simulink model "DR_Telemedicine_Screening_Workflow"  (R2024b)
settings: Solver=VariableStepAuto  StartTime=0.0  StopTime=28800  RelTol=1e-3
undefined symbols (not defined in the file): m, n
settings Model: Creator=amrut  LastModifiedBy=amrut

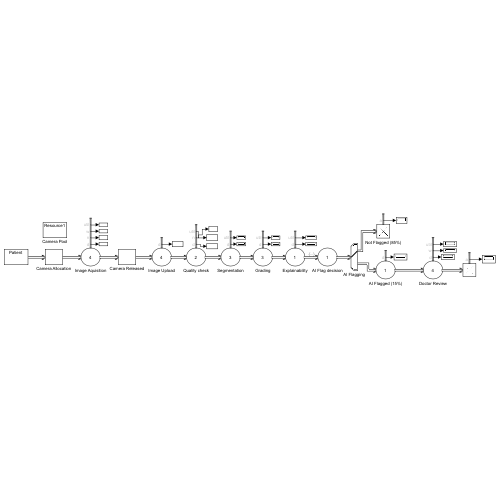
[thumbnail: Simulink's stored preview of the top-level diagram]
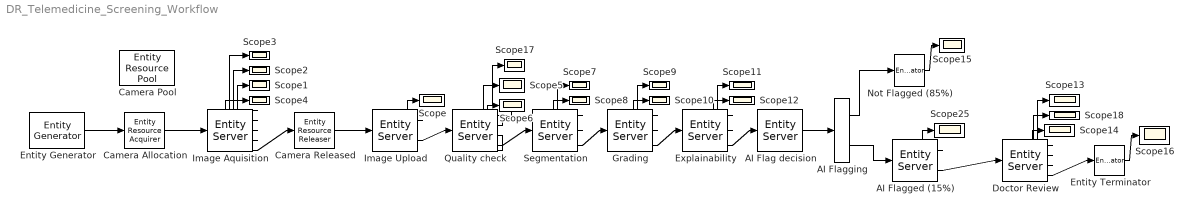
== system DR_Telemedicine_Screening_Workflow ==
  AI Flag decision : EntityServer  InputPortMessageModes=m  OutputPortMessageModes=m  Capacity=1  EntryAction=|
      | if rand < 0.15
      |     entity.Attribute1 = 2;
      | else
      |     entity.Attribute1 = 1;
      | end
  AI Flagged (15%) : EntityServer  InputPortMessageModes=m  OutputPortMessageModes=n,m  Capacity=1  NumberEntitiesDeparted=on
      settings: OutputPortMap=o0,o9
  AI Flagging : EntityOutputSwitch  InputPortMessageModes=m  OutputPortMessageModes=m,m  SwitchingCriterion=From attribute  SwitchAttributeName=Attribute1
  Camera Allocation : EntityResourceAcquirer  InputPortMessageModes=m  OutputPortMessageModes=m  NumberWaitingEntities=inf
      settings: OutputPortMap=o3
  Camera Pool : EntityResourcePool  ResourceAmount=4
  Camera Released : EntityResourceReleaser  InputPortMessageModes=m  OutputPortMessageModes=m  ResourceToRelease=Selected  ResourceAmount=1
  Doctor Review : EntityServer  InputPortMessageModes=m  OutputPortMessageModes=n,n,n,m  Capacity=4  ServiceTimeValue=900  NumberEntitiesDeparted=on  AverageWait=on  Utilization=on
      settings: OutputPortMap=o0,o4,o5,o9
  Entity Generator : EntityGenerator  OutputPortMessageModes=m  Period=86.49  EntityType=Structured  EntityTypeName=Patient
  Entity Terminator : EntityTerminator  InputPortMessageModes=m  NumberEntitiesArrived=on
      settings: OutputPortMap=o0
  Explainability : EntityServer  InputPortMessageModes=m  OutputPortMessageModes=n,n,m  Capacity=1  ServiceTimeValue=30  NumberEntitiesDeparted=on  Utilization=on
      settings: OutputPortMap=o0,o5,o9
  Grading : EntityServer  InputPortMessageModes=m  OutputPortMessageModes=n,n,m  Capacity=3  ServiceTimeValue=60  NumberEntitiesDeparted=on  Utilization=on
      settings: OutputPortMap=o0,o5,o9
  Image Aquisition : EntityServer  InputPortMessageModes=m  OutputPortMessageModes=n,n,n,n,m  Capacity=4  ServiceTimeValue=300  NumberEntitiesDeparted=on  NumberEntitiesInBlock=on  AverageWait=on  Utilization=on
      settings: OutputPortMap=o0,o1,o4,o5,o9
  Image Upload : EntityServer  InputPortMessageModes=m  OutputPortMessageModes=n,m  Capacity=4  ServiceTimeValue=4  NumberEntitiesDeparted=on
      settings: OutputPortMap=o0,o9
  Not Flagged (85%) : EntityTerminator  InputPortMessageModes=m  NumberEntitiesArrived=on
      settings: OutputPortMap=o0
  Quality check : EntityServer  InputPortMessageModes=m  OutputPortMessageModes=n,n,n,m  Capacity=2  ServiceTimeValue=30  NumberEntitiesDeparted=on  NumberEntitiesInBlock=on  Utilization=on
      settings: OutputPortMap=o0,o1,o5,o9
  Scope{,1..18,25} (20 alike) : Scope
  Segmentation : EntityServer  InputPortMessageModes=m  OutputPortMessageModes=n,n,m  Capacity=3  ServiceTimeValue=90  NumberEntitiesDeparted=on  Utilization=on
      settings: OutputPortMap=o0,o5,o9
  wires:
  Entity Generator/1 -> Camera Allocation/1
  Camera Allocation/1 -> Image Aquisition/1
  Image Aquisition/5 -> Camera Released/1
  Image Aquisition/2 -> Scope1/1
  Image Aquisition/3 -> Scope2/1
  Image Aquisition/4 -> Scope3/1
  Image Aquisition/1 -> Scope4/1
  Camera Released/1 -> Image Upload/1
  Image Upload/2 -> Quality check/1
  Image Upload/1 -> Scope/1
  Quality check/1 -> Scope6/1
  Quality check/3 -> Scope5/1
  Quality check/4 -> Segmentation/1
  Segmentation/3 -> Grading/1
  Grading/3 -> Explainability/1
  AI Flagging/1 -> Not Flagged (85%)/1
  AI Flagging/2 -> AI Flagged (15%)/1
  Doctor Review/4 -> Entity Terminator/1
  Segmentation/2 -> Scope7/1
  Segmentation/1 -> Scope8/1
  Grading/2 -> Scope9/1
  Grading/1 -> Scope10/1
  Explainability/2 -> Scope11/1
  Explainability/1 -> Scope12/1
  Doctor Review/3 -> Scope13/1
  Doctor Review/1 -> Scope14/1
  Explainability/3 -> AI Flag decision/1
  AI Flag decision/1 -> AI Flagging/1
  Not Flagged (85%)/1 -> Scope15/1
  Entity Terminator/1 -> Scope16/1
  Quality check/2 -> Scope17/1
  Doctor Review/2 -> Scope18/1
  AI Flagged (15%)/1 -> Scope25/1
  AI Flagged (15%)/2 -> Doctor Review/1
